simulink model "DOF_Model"  (R2025b)
settings: Solver=VariableStepAuto  StartTime=0.0  StopTime=5*60  RelTol=1e-3
model workspace (MAT data in the model file):
  u = [0; -0.1; 0; 0; 0.08]
undefined symbols (not defined in the file or in its folder): Nonlinear_6DOF_Model
settings Model: Creator=haria  LastModifiedBy=anwak

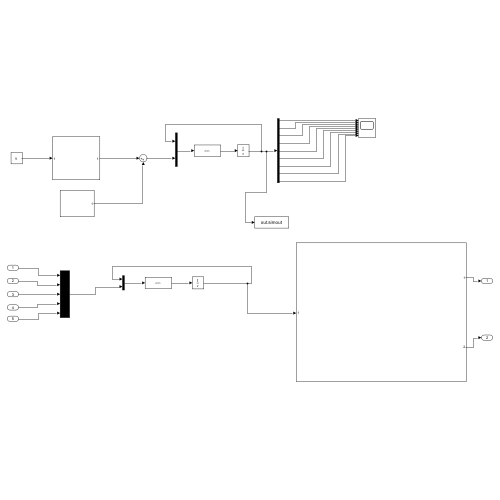
[thumbnail: Simulink's stored preview of the top-level diagram]
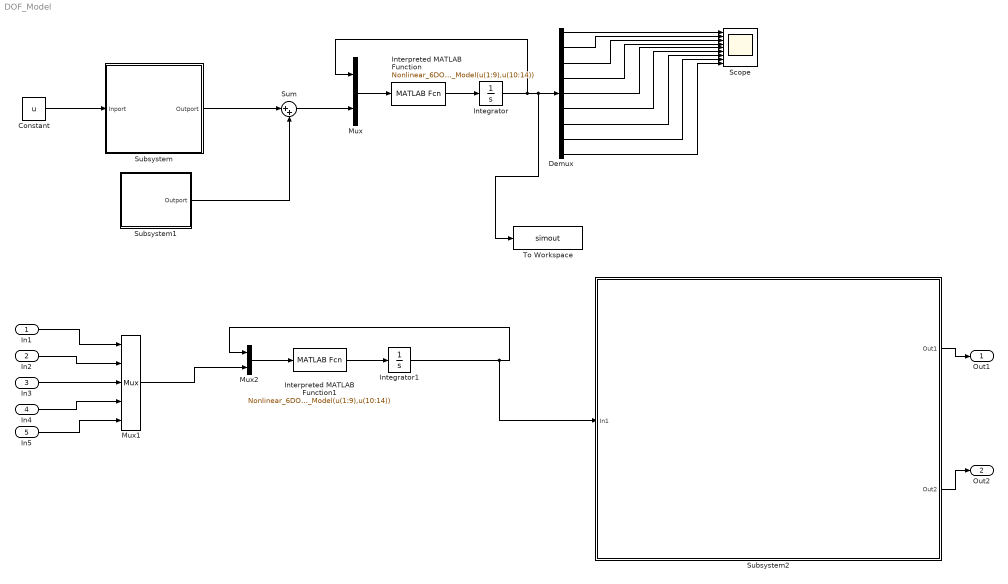
== system DOF_Model ==
  In1 : Inport
  In2 : Inport  Port=2
  In3 : Inport  Port=3
  In4 : Inport  Port=4
  In5 : Inport  Port=5
  Constant : Constant  Value=u
  Demux : Demux  Outputs=9
  Integrator : Integrator  InitialCondition=[85; 0;0;0;0;0;0;0.1;0]
  Integrator1 : Integrator  InitialCondition=[85; 0;0;0;0;0;0;0.1;0]
  Interpreted MATLAB Function : MATLABFcn  MATLABFcn=Nonlinear_6DOF_Model(u(1:9),u(10:14))
  Interpreted MATLAB Function1 : MATLABFcn  MATLABFcn=Nonlinear_6DOF_Model(u(1:9),u(10:14))
  Mux : Mux  Inputs=2
  Mux1 : Mux  Inputs=5
  Mux2 : Mux  Inputs=2
  Scope : Scope  NumInputPorts=9
      settings: ActiveDisplayYMinimum=80.286358891438638  ActiveDisplayYMaximum=94.849130364102123
  Subsystem : Subsystem
  Subsystem1 : Subsystem
  Subsystem2 : Subsystem
  Sum : Sum  Inputs=|++
  To Workspace : ToWorkspace  VariableName=simout  SaveFormat=Timeseries  SampleTime=-1
  Out1 : Outport
  Out2 : Outport  Port=2
  wires:
  Constant/1 -> Subsystem/1(Inport)
  Subsystem/1(Outport) -> Sum/1
  Subsystem1/1(Outport) -> Sum/2
  Sum/1 -> Mux/2
  Mux/1 -> Interpreted MATLAB Function/1
  Interpreted MATLAB Function/1 -> Integrator/1
  Integrator/1 -> Mux/1, To Workspace/1, Demux/1
  Demux/1 -> Scope/1
  Demux/2 -> Scope/2
  Demux/3 -> Scope/3
  Demux/4 -> Scope/4
  Demux/5 -> Scope/5
  Demux/6 -> Scope/6
  Demux/7 -> Scope/7
  Demux/8 -> Scope/8
  Demux/9 -> Scope/9
  In1/1 -> Mux1/1
  In2/1 -> Mux1/2
  In3/1 -> Mux1/3
  In4/1 -> Mux1/4
  In5/1 -> Mux1/5
  Mux1/1 -> Mux2/2
  Mux2/1 -> Interpreted MATLAB Function1/1
  Interpreted MATLAB Function1/1 -> Integrator1/1
  Integrator1/1 -> Subsystem2/1(In1), Mux2/1
  Subsystem2/1(Out1) -> Out1/1
  Subsystem2/2(Out2) -> Out2/1

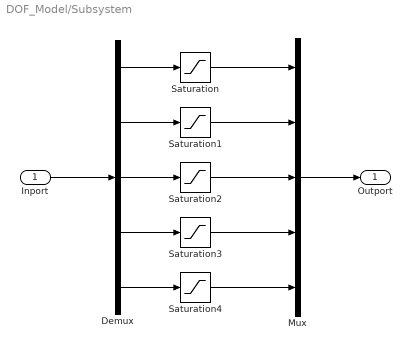
== system DOF_Model/Subsystem ==
  Inport : Inport
  Demux : Demux  Outputs=5
  Mux : Mux  Inputs=5
  Saturation : Saturate  UpperLimit=25*(pi/180)  LowerLimit=-25*(pi/180)
  Saturation1 : Saturate  UpperLimit=10*(pi/180)  LowerLimit=-25*(pi/180)
  Saturation2 : Saturate  UpperLimit=30*(pi/180)  LowerLimit=-30*(pi/180)
  Saturation3 : Saturate  UpperLimit=10*(pi/180)  LowerLimit=0.5*(pi/180)
  Saturation4 : Saturate  UpperLimit=10*(pi/180)  LowerLimit=0.5*(pi/180)
  Outport : Outport
  wires:
  Saturation/1 -> Mux/1
  Demux/3 -> Saturation2/1
  Demux/5 -> Saturation4/1
  Demux/2 -> Saturation1/1
  Saturation2/1 -> Mux/3
  Saturation3/1 -> Mux/4
  Demux/1 -> Saturation/1
  Demux/4 -> Saturation3/1
  Mux/1 -> Outport/1
  Saturation4/1 -> Mux/5
  Inport/1 -> Demux/1
  Saturation1/1 -> Mux/2

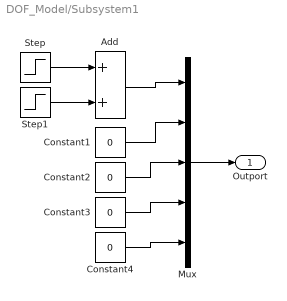
== system DOF_Model/Subsystem1 ==
  Add : Sum
  Constant{1..4} (4 alike) : Constant  Value=0
  Mux : Mux  Inputs=5
  Step : Step  Time=30  After=5*(pi/180)  SampleTime=0
  Step1 : Step  Time=32  After=-5*(pi/180)  SampleTime=0
  Outport : Outport
  wires:
  Constant3/1 -> Mux/4
  Constant1/1 -> Mux/2
  Constant2/1 -> Mux/3
  Step1/1 -> Add/2
  Add/1 -> Mux/1
  Mux/1 -> Outport/1
  Step/1 -> Add/1
  Constant4/1 -> Mux/5

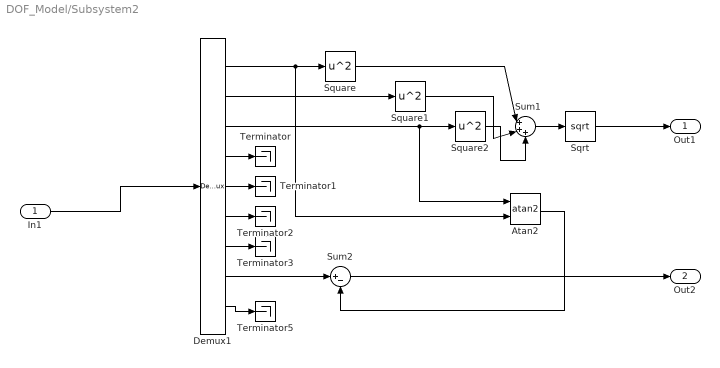
== system DOF_Model/Subsystem2 ==
  In1 : Inport
  Atan2 : Trigonometry  Operator=atan2
  Demux1 : Demux  Outputs=9
  Sqrt : Sqrt
  Square : Math  Operator=square
  Square1 : Math  Operator=square
  Square2 : Math  Operator=square
  Sum1 : Sum  Inputs=|+++
  Sum2 : Sum  Inputs=|+-
  Terminator{,1..3,5} (5 alike) : Terminator
  Out1 : Outport
  Out2 : Outport  Port=2
  wires:
  Demux1/1 -> Atan2/2, Square/1
  Demux1/8 -> Sum2/1
  Demux1/7 -> Terminator3/1
  Demux1/6 -> Terminator2/1
  Square2/1 -> Sum1/3
  Square1/1 -> Sum1/2
  Sum1/1 -> Sqrt/1
  Demux1/3 -> Atan2/1, Square2/1
  Demux1/2 -> Square1/1
  Demux1/4 -> Terminator/1
  Sqrt/1 -> Out1/1
  Demux1/9 -> Terminator5/1
  Square/1 -> Sum1/1
  Demux1/5 -> Terminator1/1
  Atan2/1 -> Sum2/2
  Sum2/1 -> Out2/1
  In1/1 -> Demux1/1
